simulink model "e4_tank_reactor_no_error_dyn"  (R2020a)
settings: Solver=FixedStepAuto  StartTime=0.0  StopTime=options.T_train  FixedStep=options.dt  RelTol=1e-3
PreLoadFcn:
  | load e4_PIDGainSchedExample.mat
model workspace (MAT data in the model file):
  op_snapshot1 : handle (value not decoded)
values from neighbouring files (symbols this model uses):
  C = [2 3 4 5 6 7 8 9]    [e4_PIDGainSchedExample.mat]
undefined symbols (not defined in the file or in its folder): Controllers, D, I, N, options, P, sigbuilder_block
libraries: neural x132, simulink x2, simulink_need_slupdate x1
(part 2 of 6)

== system e4_tank_reactor_no_error_dyn/NN/Layer 1/Delays 1 ==
  "p{1}" : Inport  PortDimensions=8
      mask Display: e = 0.06;c1 = [120 230 180]/255;c2 = ([120 230 180]+0)/(256+128);c3 = ([120 230 180]+128)/(256+128);patch([0 1 1 0],[0 0 1 1],c1);patch([0 1 1 1-e 1-e 0+e],[0 0 1 1-e 0+e 0+e],c2);patch([0 0 1 1-e 0+e 0+e],[0 1 1 1-e 1-e 0+e],c3);plot([0 1 1 0 0],[0 0 1 1 0]);
  mux : Mux  Inputs=1
      mask Display: e = 0.06;c1 = [120 150 230]/255;c2 = ([120 150 230]+0)/383;c3 = ([120 150 230]+128)/383;patch([0 1 1 0],[0 0 1 1],c1);patch([0 1 1 1-e 1-e 0+e],[0 0 1 1-e 0+e 0+e],c2);patch([0 0 1 1-e 0+e 0+e],[0 1 1 1-e 1-e 0+e],c3);plot([0 1 1 0 0],[0 0 1 1 0]);disp('Mux')
  "pd{1,1}" : Outport
      mask Display: e = 0.06;c1 = [120 230 180]/255;c2 = ([120 230 180]+0)/(256+128);c3 = ([120 230 180]+128)/(256+128);patch([0 1 1 0],[0 0 1 1],c1);patch([0 1 1 1-e 1-e 0+e],[0 0 1 1-e 0+e 0+e],c2);patch([0 0 1 1-e 0+e 0+e],[0 1 1 1-e 1-e 0+e],c3);plot([0 1 1 0 0],[0 0 1 1 0]);
  wires:
  "p{1}"/1 -> mux/1
  mux/1 -> "pd{1,1}"/1

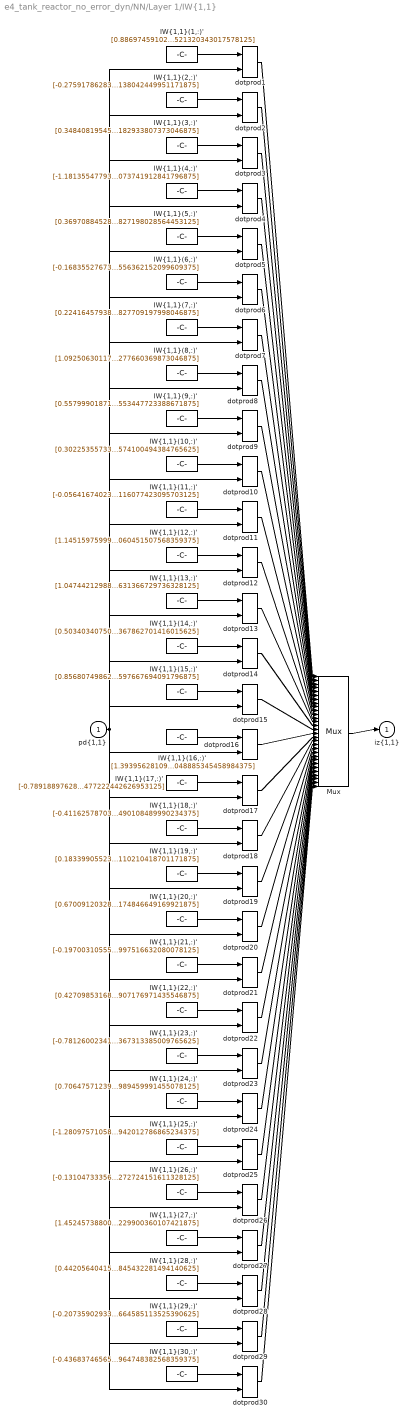
== system e4_tank_reactor_no_error_dyn/NN/Layer 1/IW{1,1} ==
  "pd{1,1}" : Inport  PortDimensions=8
      mask Display: e = 0.06;c1 = [120 230 180]/255;c2 = ([120 230 180]+0)/(256+128);c3 = ([120 230 180]+128)/(256+128);patch([0 1 1 0],[0 0 1 1],c1);patch([0 1 1 1-e 1-e 0+e],[0 0 1 1-e 0+e 0+e],c2);patch([0 0 1 1-e 0+e 0+e],[0 1 1 1-e 1-e 0+e],c3);plot([0 1 1 0 0],[0 0 1 1 0]);
  "IW{1,1}(1,:)'" : Constant  Value=[0.8869745910205413252924699918366968631744384765625;-0.003402523557962419502309625585212415899150073528289794921875;0.167531227865286069800276891328394412994384765625;0.10286305198869487298463099023138056509196758270263671875;-0.71703402880353894754961174839991144835948944091796875;-1.2912603656687069442199344848631881177425384521484375;0.9076414187719077375504639348946511745452880859375;0.424730339919138721871405550700728781521320343017578125]
      mask Display: e = 0.06;c1 = [120 150 230]/255;c2 = ([120 150 230]+0)/383;c3 = ([120 150 230]+128)/383;patch([0 1 1 0],[0 0 1 1],c1);patch([0 1 1 1-e 1-e 0+e],[0 0 1 1-e 0+e 0+e],c2);patch([0 0 1 1-e 0+e 0+e],[0 1 1 1-e 1-e 0+e],c3);plot([0 1 1 0 0],[0 0 1 1 0]);disp('Weights');
  "IW{1,1}(10,:)'" : Constant  Value=[0.302253557331712829903125339114922098815441131591796875;-1.9983086879888884990208453018567524850368499755859375;1.273941183184043257625717160408385097980499267578125;-1.018922795975827799708213206031359732151031494140625;2.4603325055853648706261083134450018405914306640625;-0.7659472736172781015540067528490908443927764892578125;-0.70371299108074636396992218578816391527652740478515625;0.12058703123603677076491891284604207612574100494384765625]
      mask Display: e = 0.06;c1 = [120 150 230]/255;c2 = ([120 150 230]+0)/383;c3 = ([120 150 230]+128)/383;patch([0 1 1 0],[0 0 1 1],c1);patch([0 1 1 1-e 1-e 0+e],[0 0 1 1-e 0+e 0+e],c2);patch([0 0 1 1-e 0+e 0+e],[0 1 1 1-e 1-e 0+e],c3);plot([0 1 1 0 0],[0 0 1 1 0]);disp('Weights');
  "IW{1,1}(11,:)'" : Constant  Value=[-0.056416740236481743853147463596542365849018096923828125;1.88817871488456301420910676824860274791717529296875;-0.2850288013275081855368853211984969675540924072265625;-0.60909058798571746873307120040408335626125335693359375;-1.1722779325389647286925765001797117292881011962890625;2.0040908100766454680297101731412112712860107421875;0.526873639458410369940111195319332182407379150390625;-0.92068711979477424467432911114883609116077423095703125]
      mask Display: e = 0.06;c1 = [120 150 230]/255;c2 = ([120 150 230]+0)/383;c3 = ([120 150 230]+128)/383;patch([0 1 1 0],[0 0 1 1],c1);patch([0 1 1 1-e 1-e 0+e],[0 0 1 1-e 0+e 0+e],c2);patch([0 0 1 1-e 0+e 0+e],[0 1 1 1-e 1-e 0+e],c3);plot([0 1 1 0 0],[0 0 1 1 0]);disp('Weights');
  "IW{1,1}(12,:)'" : Constant  Value=[1.14515975999364894022392036276869475841522216796875;-0.8542807808416206238888435109402053058147430419921875;1.066709048371362822393848546198569238185882568359375;0.377840995831276560412703702240833081305027008056640625;-1.020663060599571014819275660556741058826446533203125;-0.76558848030476622792406260487041436135768890380859375;0.7064741359778070606267874609329737722873687744140625;-0.6900660399931834998454860397032462060451507568359375]
      mask Display: e = 0.06;c1 = [120 150 230]/255;c2 = ([120 150 230]+0)/383;c3 = ([120 150 230]+128)/383;patch([0 1 1 0],[0 0 1 1],c1);patch([0 1 1 1-e 1-e 0+e],[0 0 1 1-e 0+e 0+e],c2);patch([0 0 1 1-e 0+e 0+e],[0 1 1 1-e 1-e 0+e],c3);plot([0 1 1 0 0],[0 0 1 1 0]);disp('Weights');
  "IW{1,1}(13,:)'" : Constant  Value=[1.04744212988422180643510728259570896625518798828125;-1.2053415482433142980056572923786006867885589599609375;-0.7225578173341260512785311220795847475528717041015625;-0.584831305619675223539388753124512732028961181640625;0.85698675098009668982257380775990895926952362060546875;-0.71145783550227281732958317661541514098644256591796875;-0.29166444409964886741448708562529645860195159912109375;-0.39113888775617511317506114210118539631366729736328125]
      mask Display: e = 0.06;c1 = [120 150 230]/255;c2 = ([120 150 230]+0)/383;c3 = ([120 150 230]+128)/383;patch([0 1 1 0],[0 0 1 1],c1);patch([0 1 1 1-e 1-e 0+e],[0 0 1 1-e 0+e 0+e],c2);patch([0 0 1 1-e 0+e 0+e],[0 1 1 1-e 1-e 0+e],c3);plot([0 1 1 0 0],[0 0 1 1 0]);disp('Weights');
  "IW{1,1}(14,:)'" : Constant  Value=[0.503403407506826994222137727774679660797119140625;-0.54357297238896240543226667796261608600616455078125;0.9874634317779336090126207636785693466663360595703125;0.033746523035958576886006454742528148926794528961181640625;-0.254811710231782118096788281036424450576305389404296875;0.86220415793024252071319324386422522366046905517578125;-0.83902536220982260051215462226537056267261505126953125;0.65023292766698459477225924274534918367862701416015625]
      mask Display: e = 0.06;c1 = [120 150 230]/255;c2 = ([120 150 230]+0)/383;c3 = ([120 150 230]+128)/383;patch([0 1 1 0],[0 0 1 1],c1);patch([0 1 1 1-e 1-e 0+e],[0 0 1 1-e 0+e 0+e],c2);patch([0 0 1 1-e 0+e 0+e],[0 1 1 1-e 1-e 0+e],c3);plot([0 1 1 0 0],[0 0 1 1 0]);disp('Weights');
  "IW{1,1}(15,:)'" : Constant  Value=[0.8568074986297740114338239436619915068149566650390625;-0.683506818415545058797988531296141445636749267578125;0.90244622966523613261102809701696969568729400634765625;-1.944132599731748012317211760091595351696014404296875;-0.58519215004215630049344554208801127970218658447265625;0.32903336516029302316610483103431761264801025390625;0.65754868586560533127993721791426651179790496826171875;-0.99959059893120627560136881584185175597667694091796875]
      mask Display: e = 0.06;c1 = [120 150 230]/255;c2 = ([120 150 230]+0)/383;c3 = ([120 150 230]+128)/383;patch([0 1 1 0],[0 0 1 1],c1);patch([0 1 1 1-e 1-e 0+e],[0 0 1 1-e 0+e 0+e],c2);patch([0 0 1 1-e 0+e 0+e],[0 1 1 1-e 1-e 0+e],c3);plot([0 1 1 0 0],[0 0 1 1 0]);disp('Weights');
  "IW{1,1}(16,:)'" : Constant  Value=[1.3939562810990129282373573005315847694873809814453125;1.0876382522002334685140567671624012291431427001953125;1.2710703159320801969300873679458163678646087646484375;-1.17347063100059489926252354052849113941192626953125;1.10341011023059021312064942321740090847015380859375;-0.316324187931432410092469353912747465074062347412109375;-0.7059769814258747278046257633832283318042755126953125;0.18481149462138490857654460342018865048885345458984375]
      mask Display: e = 0.06;c1 = [120 150 230]/255;c2 = ([120 150 230]+0)/383;c3 = ([120 150 230]+128)/383;patch([0 1 1 0],[0 0 1 1],c1);patch([0 1 1 1-e 1-e 0+e],[0 0 1 1-e 0+e 0+e],c2);patch([0 0 1 1-e 0+e 0+e],[0 1 1 1-e 1-e 0+e],c3);plot([0 1 1 0 0],[0 0 1 1 0]);disp('Weights');
  "IW{1,1}(17,:)'" : Constant  Value=[-0.78918897628251272191590715010534040629863739013671875;-0.69345544068538178539284899670747108757495880126953125;1.133331701461687490706253811367787420749664306640625;0.481227638616822994688249082173570059239864349365234375;1.394399245993624969486290865461342036724090576171875;0.7686987843847490342596984191914089024066925048828125;1.4818227960370886631125131316366605460643768310546875;-0.125485665132124613041497696031001396477222442626953125]
      mask Display: e = 0.06;c1 = [120 150 230]/255;c2 = ([120 150 230]+0)/383;c3 = ([120 150 230]+128)/383;patch([0 1 1 0],[0 0 1 1],c1);patch([0 1 1 1-e 1-e 0+e],[0 0 1 1-e 0+e 0+e],c2);patch([0 0 1 1-e 0+e 0+e],[0 1 1 1-e 1-e 0+e],c3);plot([0 1 1 0 0],[0 0 1 1 0]);disp('Weights');
  "IW{1,1}(18,:)'" : Constant  Value=[-0.4116257870393840168077304042526520788669586181640625;0.342402945255573187832709436406730674207210540771484375;0.6993052671719846014042332171811722218990325927734375;-0.04069640465013980856756603543544770218431949615478515625;0.060718970322058203603621251431832206435501575469970703125;-1.4315780103489730290533543666242621839046478271484375;0.746726210319609950971653233864344656467437744140625;-0.66922398088218082445877143982215784490108489990234375]
      mask Display: e = 0.06;c1 = [120 150 230]/255;c2 = ([120 150 230]+0)/383;c3 = ([120 150 230]+128)/383;patch([0 1 1 0],[0 0 1 1],c1);patch([0 1 1 1-e 1-e 0+e],[0 0 1 1-e 0+e 0+e],c2);patch([0 0 1 1-e 0+e 0+e],[0 1 1 1-e 1-e 0+e],c3);plot([0 1 1 0 0],[0 0 1 1 0]);disp('Weights');
  "IW{1,1}(19,:)'" : Constant  Value=[0.18339905523404398390852065858780406415462493896484375;1.5668662807207969223100008093751966953277587890625;-0.0268049996970174918275997555383582948707044124603271484375;0.07428825726819134056544413624578737653791904449462890625;-1.878491586774890809152793735847808420658111572265625;1.1916603403785341885878779066842980682849884033203125;1.672592346593904988338863404351286590099334716796875;-0.25617012853654486104204579532961361110210418701171875]
      mask Display: e = 0.06;c1 = [120 150 230]/255;c2 = ([120 150 230]+0)/383;c3 = ([120 150 230]+128)/383;patch([0 1 1 0],[0 0 1 1],c1);patch([0 1 1 1-e 1-e 0+e],[0 0 1 1-e 0+e 0+e],c2);patch([0 0 1 1-e 0+e 0+e],[0 1 1 1-e 1-e 0+e],c3);plot([0 1 1 0 0],[0 0 1 1 0]);disp('Weights');
  "IW{1,1}(2,:)'" : Constant  Value=[-0.27591786283207986318899429534212686121463775634765625;3.196411383092458091681464793509803712368011474609375;-1.0488445244355248942014213753282092511653900146484375;0.320146632870869807252489636084646917879581451416015625;-0.76571063454435772666073489745031110942363739013671875;-0.055011350027142767726839878150713047944009304046630859375;1.202802065550638843660635757260024547576904296875;-0.383647276981947171758946524278144352138042449951171875]
      mask Display: e = 0.06;c1 = [120 150 230]/255;c2 = ([120 150 230]+0)/383;c3 = ([120 150 230]+128)/383;patch([0 1 1 0],[0 0 1 1],c1);patch([0 1 1 1-e 1-e 0+e],[0 0 1 1-e 0+e 0+e],c2);patch([0 0 1 1-e 0+e 0+e],[0 1 1 1-e 1-e 0+e],c3);plot([0 1 1 0 0],[0 0 1 1 0]);disp('Weights');
  "IW{1,1}(20,:)'" : Constant  Value=[0.67009120328841598190905415322049520909786224365234375;-0.5515720185612804637997896861634217202663421630859375;-0.55267982206462662464474533408065326511859893798828125;-0.6448735709813189220795948131126351654529571533203125;0.06989978721913596426684733842193963937461376190185546875;-1.6288120176144247341909476745058782398700714111328125;0.779509281707432055696926909149624407291412353515625;1.310159712789221497786229519988410174846649169921875]
      mask Display: e = 0.06;c1 = [120 150 230]/255;c2 = ([120 150 230]+0)/383;c3 = ([120 150 230]+128)/383;patch([0 1 1 0],[0 0 1 1],c1);patch([0 1 1 1-e 1-e 0+e],[0 0 1 1-e 0+e 0+e],c2);patch([0 0 1 1-e 0+e 0+e],[0 1 1 1-e 1-e 0+e],c3);plot([0 1 1 0 0],[0 0 1 1 0]);disp('Weights');
  "IW{1,1}(21,:)'" : Constant  Value=[-0.1970031055596904445703643204979016445577144622802734375;-1.563987121958660964082810096442699432373046875;0.61059106825549569474986810746486298739910125732421875;1.031098034825259635027805416029877960681915283203125;0.56196026107034768859449513911386020481586456298828125;-1.9981853523962189722595894636469893157482147216796875;1.0888860789131200590418302454054355621337890625;-0.09361921948207392596419396113560651428997516632080078125]
      mask Display: e = 0.06;c1 = [120 150 230]/255;c2 = ([120 150 230]+0)/383;c3 = ([120 150 230]+128)/383;patch([0 1 1 0],[0 0 1 1],c1);patch([0 1 1 1-e 1-e 0+e],[0 0 1 1-e 0+e 0+e],c2);patch([0 0 1 1-e 0+e 0+e],[0 1 1 1-e 1-e 0+e],c3);plot([0 1 1 0 0],[0 0 1 1 0]);disp('Weights');
  "IW{1,1}(22,:)'" : Constant  Value=[0.427098531684761584248377630501636303961277008056640625;1.6076476568007012080130380127229727804660797119140625;-1.1014857891164815395512732720817439258098602294921875;0.36149790428804406960949791027815081179141998291015625;-0.248586804369456626506718066593748517334461212158203125;-0.69684275999031886072998531744815409183502197265625;-0.286841168321181394507135564708732999861240386962890625;0.422714361893740953046716413155081681907176971435546875]
      mask Display: e = 0.06;c1 = [120 150 230]/255;c2 = ([120 150 230]+0)/383;c3 = ([120 150 230]+128)/383;patch([0 1 1 0],[0 0 1 1],c1);patch([0 1 1 1-e 1-e 0+e],[0 0 1 1-e 0+e 0+e],c2);patch([0 0 1 1-e 0+e 0+e],[0 1 1 1-e 1-e 0+e],c3);plot([0 1 1 0 0],[0 0 1 1 0]);disp('Weights');
  "IW{1,1}(23,:)'" : Constant  Value=[-0.78126002341995481881298246662481687963008880615234375;-1.169284710329954624086212788824923336505889892578125;1.166017240859436920885627841926179826259613037109375;-0.8507388975249752238738665255368687212467193603515625;1.191358648701899891619859772617928683757781982421875;0.63702009366910161691777148007531650364398956298828125;0.74006431103171299579202013774192892014980316162109375;0.07772625224719166558973171277102665044367313385009765625]
      mask Display: e = 0.06;c1 = [120 150 230]/255;c2 = ([120 150 230]+0)/383;c3 = ([120 150 230]+128)/383;patch([0 1 1 0],[0 0 1 1],c1);patch([0 1 1 1-e 1-e 0+e],[0 0 1 1-e 0+e 0+e],c2);patch([0 0 1 1-e 0+e 0+e],[0 1 1 1-e 1-e 0+e],c3);plot([0 1 1 0 0],[0 0 1 1 0]);disp('Weights');
  "IW{1,1}(24,:)'" : Constant  Value=[0.7064757123964204854615900330827571451663970947265625;-1.18446852299836802302479554782621562480926513671875;0.8255008023140779638282538144267164170742034912109375;-1.131032706182091285285196136101149022579193115234375;-0.09862722601019034696090415081926039420068264007568359375;0.373718657230955653147930206614546477794647216796875;-0.238682435995127895100864634514437057077884674072265625;0.7577262920549394653590979942237026989459991455078125]
      mask Display: e = 0.06;c1 = [120 150 230]/255;c2 = ([120 150 230]+0)/383;c3 = ([120 150 230]+128)/383;patch([0 1 1 0],[0 0 1 1],c1);patch([0 1 1 1-e 1-e 0+e],[0 0 1 1-e 0+e 0+e],c2);patch([0 0 1 1-e 0+e 0+e],[0 1 1 1-e 1-e 0+e],c3);plot([0 1 1 0 0],[0 0 1 1 0]);disp('Weights');
  "IW{1,1}(25,:)'" : Constant  Value=[-1.2809757105870402948966102485428564250469207763671875;-0.82852550051283835319537729446892626583576202392578125;-0.32970505738248034877102554673911072313785552978515625;-0.279935523019308851733200071976170875132083892822265625;-1.055968298065763644189019032637588679790496826171875;0.704919073979582311295644103665836155414581298828125;-0.435018707569000684376447907197871245443820953369140625;0.7523081434708822623491641934379003942012786865234375]
      mask Display: e = 0.06;c1 = [120 150 230]/255;c2 = ([120 150 230]+0)/383;c3 = ([120 150 230]+128)/383;patch([0 1 1 0],[0 0 1 1],c1);patch([0 1 1 1-e 1-e 0+e],[0 0 1 1-e 0+e 0+e],c2);patch([0 0 1 1-e 0+e 0+e],[0 1 1 1-e 1-e 0+e],c3);plot([0 1 1 0 0],[0 0 1 1 0]);disp('Weights');
  "IW{1,1}(26,:)'" : Constant  Value=[-0.13104733356740727590050710205105133354663848876953125;2.32195529483453189101282987394370138645172119140625;-1.88567524333584923823536882991902530193328857421875;0.6858958644523547310001276855473406612873077392578125;-0.50214888361890064327752725148457102477550506591796875;-1.2241599972289074482745263594551943242549896240234375;0.34451596634661718621117643124307505786418914794921875;-0.1756704889982736716991240655261208303272724151611328125]
      mask Display: e = 0.06;c1 = [120 150 230]/255;c2 = ([120 150 230]+0)/383;c3 = ([120 150 230]+128)/383;patch([0 1 1 0],[0 0 1 1],c1);patch([0 1 1 1-e 1-e 0+e],[0 0 1 1-e 0+e 0+e],c2);patch([0 0 1 1-e 0+e 0+e],[0 1 1 1-e 1-e 0+e],c3);plot([0 1 1 0 0],[0 0 1 1 0]);disp('Weights');
  "IW{1,1}(27,:)'" : Constant  Value=[1.452457388008406180546217001392506062984466552734375;-1.172610436821962753839443394099362194538116455078125;-0.9004330461382306083351068082265555858612060546875;1.208817515055535363188710107351653277873992919921875;-1.5350383119922803576429259919677861034870147705078125;-1.2583216228706193273723101810901425778865814208984375;0.270644327489568625733085127649246715009212493896484375;-0.311405295052269159850055757488007657229900360107421875]
      mask Display: e = 0.06;c1 = [120 150 230]/255;c2 = ([120 150 230]+0)/383;c3 = ([120 150 230]+128)/383;patch([0 1 1 0],[0 0 1 1],c1);patch([0 1 1 1-e 1-e 0+e],[0 0 1 1-e 0+e 0+e],c2);patch([0 0 1 1-e 0+e 0+e],[0 1 1 1-e 1-e 0+e],c3);plot([0 1 1 0 0],[0 0 1 1 0]);disp('Weights');
  "IW{1,1}(28,:)'" : Constant  Value=[0.442056404152748660951743886471376754343509674072265625;0.2493526475618815518853210733141168020665645599365234375;0.1181239015107082568345475692694890312850475311279296875;-0.2496322625530794370174447749377577565610408782958984375;-1.4116755942211833829702527509653009474277496337890625;-0.244632780309239461491443989871186204254627227783203125;-0.92786848745628847101585279233404435217380523681640625;0.1302999051855696921453642289634444750845432281494140625]
      mask Display: e = 0.06;c1 = [120 150 230]/255;c2 = ([120 150 230]+0)/383;c3 = ([120 150 230]+128)/383;patch([0 1 1 0],[0 0 1 1],c1);patch([0 1 1 1-e 1-e 0+e],[0 0 1 1-e 0+e 0+e],c2);patch([0 0 1 1-e 0+e 0+e],[0 1 1 1-e 1-e 0+e],c3);plot([0 1 1 0 0],[0 0 1 1 0]);disp('Weights');
  "IW{1,1}(29,:)'" : Constant  Value=[-0.2073590293315980270794085527086281217634677886962890625;-1.261453485543998720430636240052990615367889404296875;0.417145317623059508349570023710839450359344482421875;0.4401304305971904806682459820876829326152801513671875;0.8012367360713794628424011534661985933780670166015625;0.93557485529794803813530279512633569538593292236328125;0.36557613193985805111196896177716553211212158203125;-1.159475113688609670958840069943107664585113525390625]
      mask Display: e = 0.06;c1 = [120 150 230]/255;c2 = ([120 150 230]+0)/383;c3 = ([120 150 230]+128)/383;patch([0 1 1 0],[0 0 1 1],c1);patch([0 1 1 1-e 1-e 0+e],[0 0 1 1-e 0+e 0+e],c2);patch([0 0 1 1-e 0+e 0+e],[0 1 1 1-e 1-e 0+e],c3);plot([0 1 1 0 0],[0 0 1 1 0]);disp('Weights');
  "IW{1,1}(3,:)'" : Constant  Value=[0.348408195456650859878067194586037658154964447021484375;0.13128979584945010827823352883569896221160888671875;-1.2462763128456197936344551635556854307651519775390625;0.8373497908577769432980630881502293050289154052734375;0.680450778974826864242686497163958847522735595703125;-0.7039887459854632378863925623591057956218719482421875;-1.1005637181368499444289454913814552128314971923828125;-0.666422487535424323823463055305182933807373046875]
      mask Display: e = 0.06;c1 = [120 150 230]/255;c2 = ([120 150 230]+0)/383;c3 = ([120 150 230]+128)/383;patch([0 1 1 0],[0 0 1 1],c1);patch([0 1 1 1-e 1-e 0+e],[0 0 1 1-e 0+e 0+e],c2);patch([0 0 1 1-e 0+e 0+e],[0 1 1 1-e 1-e 0+e],c3);plot([0 1 1 0 0],[0 0 1 1 0]);disp('Weights');
  "IW{1,1}(30,:)'" : Constant  Value=[-0.43683746565477676870870027414639480412006378173828125;0.414885905669120591543475029538967646658420562744140625;0.71161051729680802058197741644107736647129058837890625;-0.0266920397314014158640649299059077748097479343414306640625;-1.3723826044633893328494878005585633218288421630859375;-0.4296181668357093030863325111567974090576171875;-1.212987357728822157554304794757626950740814208984375;-0.67853804582980214998855217345408163964748382568359375]
      mask Display: e = 0.06;c1 = [120 150 230]/255;c2 = ([120 150 230]+0)/383;c3 = ([120 150 230]+128)/383;patch([0 1 1 0],[0 0 1 1],c1);patch([0 1 1 1-e 1-e 0+e],[0 0 1 1-e 0+e 0+e],c2);patch([0 0 1 1-e 0+e 0+e],[0 1 1 1-e 1-e 0+e],c3);plot([0 1 1 0 0],[0 0 1 1 0]);disp('Weights');
  "IW{1,1}(4,:)'" : Constant  Value=[-1.1813554779349157985990359520656056702136993408203125;1.3081343050477116651819642356713302433490753173828125;0.1111861520282881043986122904243529774248600006103515625;0.302078564819876493885431045782752335071563720703125;-1.215049696649854293895032242289744317531585693359375;-0.339238609197104412640300097336876206099987030029296875;-0.146943201435645598440515868787770159542560577392578125;0.19192274869351688693086543935351073741912841796875]
      mask Display: e = 0.06;c1 = [120 150 230]/255;c2 = ([120 150 230]+0)/383;c3 = ([120 150 230]+128)/383;patch([0 1 1 0],[0 0 1 1],c1);patch([0 1 1 1-e 1-e 0+e],[0 0 1 1-e 0+e 0+e],c2);patch([0 0 1 1-e 0+e 0+e],[0 1 1 1-e 1-e 0+e],c3);plot([0 1 1 0 0],[0 0 1 1 0]);disp('Weights');
  "IW{1,1}(5,:)'" : Constant  Value=[0.369708845289564658198600000105216167867183685302734375;-1.1370366447060458181539388533565215766429901123046875;1.3116044914015230204995532403700053691864013671875;-0.1427314167325453853063521592048346064984798431396484375;0.88665021491913320605959825115860439836978912353515625;0.87832821946413108804563307785429060459136962890625;-0.304666739704737621341479325565160252153873443603515625;-0.33909715679392082865462043628212995827198028564453125]
      mask Display: e = 0.06;c1 = [120 150 230]/255;c2 = ([120 150 230]+0)/383;c3 = ([120 150 230]+128)/383;patch([0 1 1 0],[0 0 1 1],c1);patch([0 1 1 1-e 1-e 0+e],[0 0 1 1-e 0+e 0+e],c2);patch([0 0 1 1-e 0+e 0+e],[0 1 1 1-e 1-e 0+e],c3);plot([0 1 1 0 0],[0 0 1 1 0]);disp('Weights');
  "IW{1,1}(6,:)'" : Constant  Value=[-0.1683552767320385668003979162676841951906681060791015625;1.4155439500628876903220998428878374397754669189453125;-0.3049936648618356560547226763446815311908721923828125;-0.1808735587972198910478027755743823945522308349609375;-0.93949487207675286271069126087240874767303466796875;-0.98517475915990926349508072235039435327053070068359375;0.52147568646198638742106368226814083755016326904296875;-0.4491059618427362121195756117231212556362152099609375]
      mask Display: e = 0.06;c1 = [120 150 230]/255;c2 = ([120 150 230]+0)/383;c3 = ([120 150 230]+128)/383;patch([0 1 1 0],[0 0 1 1],c1);patch([0 1 1 1-e 1-e 0+e],[0 0 1 1-e 0+e 0+e],c2);patch([0 0 1 1-e 0+e 0+e],[0 1 1 1-e 1-e 0+e],c3);plot([0 1 1 0 0],[0 0 1 1 0]);disp('Weights');
  "IW{1,1}(7,:)'" : Constant  Value=[0.2241645793824775523273018507097731344401836395263671875;1.342167864111561303985808990546502172946929931640625;-0.0032931951292033919721780055311910473392345011234283447265625;-0.52511153598029525202406375683494843542575836181640625;-1.6807771985161521488549851710558868944644927978515625;0.5566622950019202153981723313336260616779327392578125;0.719828629925344021245336989522911608219146728515625;0.10582018054103141391220077593970927409827709197998046875]
      mask Display: e = 0.06;c1 = [120 150 230]/255;c2 = ([120 150 230]+0)/383;c3 = ([120 150 230]+128)/383;patch([0 1 1 0],[0 0 1 1],c1);patch([0 1 1 1-e 1-e 0+e],[0 0 1 1-e 0+e 0+e],c2);patch([0 0 1 1-e 0+e 0+e],[0 1 1 1-e 1-e 0+e],c3);plot([0 1 1 0 0],[0 0 1 1 0]);disp('Weights');
  "IW{1,1}(8,:)'" : Constant  Value=[1.0925063011756928066375849084579385817050933837890625;-0.57675375136482198712428726139478385448455810546875;-0.4110002600985167564573430354357697069644927978515625;0.459619928994233040153716274289763532578945159912109375;-0.97175270511539835194270153806428425014019012451171875;0.48179036288909216079190400705556385219097137451171875;0.62766837769450789519254385595559142529964447021484375;-1.264282084455540466905176799627952277660369873046875]
      mask Display: e = 0.06;c1 = [120 150 230]/255;c2 = ([120 150 230]+0)/383;c3 = ([120 150 230]+128)/383;patch([0 1 1 0],[0 0 1 1],c1);patch([0 1 1 1-e 1-e 0+e],[0 0 1 1-e 0+e 0+e],c2);patch([0 0 1 1-e 0+e 0+e],[0 1 1 1-e 1-e 0+e],c3);plot([0 1 1 0 0],[0 0 1 1 0]);disp('Weights');
  "IW{1,1}(9,:)'" : Constant  Value=[0.55799901871459145485943054154631681740283966064453125;-0.2030729847481355931915203427706728689372539520263671875;1.198759729689530484364468065905384719371795654296875;-0.77633171495453290322785733224009163677692413330078125;0.1732250078450238983673870052371057681739330291748046875;-0.41468434699252465502894438031944446265697479248046875;-0.6686192894460825097979750353260897099971771240234375;0.039408810987360758104625091391426394693553447723388671875]
      mask Display: e = 0.06;c1 = [120 150 230]/255;c2 = ([120 150 230]+0)/383;c3 = ([120 150 230]+128)/383;patch([0 1 1 0],[0 0 1 1],c1);patch([0 1 1 1-e 1-e 0+e],[0 0 1 1-e 0+e 0+e],c2);patch([0 0 1 1-e 0+e 0+e],[0 1 1 1-e 1-e 0+e],c3);plot([0 1 1 0 0],[0 0 1 1 0]);disp('Weights');
  Mux : Mux  Inputs=30
      mask Display: e = 0.06;c1 = [120 150 230]/255;c2 = ([120 150 230]+0)/383;c3 = ([120 150 230]+128)/383;patch([0 1 1 0],[0 0 1 1],c1);patch([0 1 1 1-e 1-e 0+e],[0 0 1 1-e 0+e 0+e],c2);patch([0 0 1 1-e 0+e 0+e],[0 1 1 1-e 1-e 0+e],c3);plot([0 1 1 0 0],[0 0 1 1 0]);disp('Mux');
  dotprod{1..30} (30 alike) : neural/Weight Functions/dotprod
  "iz{1,1}" : Outport
      mask Display: e = 0.06;c1 = [120 230 180]/255;c2 = ([120 230 180]+0)/(256+128);c3 = ([120 230 180]+128)/(256+128);patch([0 1 1 0],[0 0 1 1],c1);patch([0 1 1 1-e 1-e 0+e],[0 0 1 1-e 0+e 0+e],c2);patch([0 0 1 1-e 0+e 0+e],[0 1 1 1-e 1-e 0+e],c3);plot([0 1 1 0 0],[0 0 1 1 0]);
  wires:
  "IW{1,1}(1,:)'"/1 -> dotprod1/1
  "pd{1,1}"/1 -> dotprod1/2, dotprod2/2, dotprod3/2, dotprod4/2, dotprod5/2, dotprod6/2, dotprod7/2, dotprod8/2, dotprod9/2, dotprod10/2, dotprod11/2, dotprod12/2, dotprod13/2, dotprod14/2, dotprod15/2, dotprod16/2, dotprod17/2, dotprod18/2, dotprod19/2, dotprod20/2, dotprod21/2, dotprod22/2, dotprod23/2, dotprod24/2, dotprod25/2, dotprod26/2, dotprod27/2, dotprod28/2, dotprod29/2, dotprod30/2
  dotprod1/1 -> Mux/1
  "IW{1,1}(2,:)'"/1 -> dotprod2/1
  dotprod2/1 -> Mux/2
  "IW{1,1}(3,:)'"/1 -> dotprod3/1
  dotprod3/1 -> Mux/3
  "IW{1,1}(4,:)'"/1 -> dotprod4/1
  dotprod4/1 -> Mux/4
  "IW{1,1}(5,:)'"/1 -> dotprod5/1
  dotprod5/1 -> Mux/5
  "IW{1,1}(6,:)'"/1 -> dotprod6/1
  dotprod6/1 -> Mux/6
  "IW{1,1}(7,:)'"/1 -> dotprod7/1
  dotprod7/1 -> Mux/7
  "IW{1,1}(8,:)'"/1 -> dotprod8/1
  dotprod8/1 -> Mux/8
  "IW{1,1}(9,:)'"/1 -> dotprod9/1
  dotprod9/1 -> Mux/9
  "IW{1,1}(10,:)'"/1 -> dotprod10/1
  dotprod10/1 -> Mux/10
  "IW{1,1}(11,:)'"/1 -> dotprod11/1
  dotprod11/1 -> Mux/11
  "IW{1,1}(12,:)'"/1 -> dotprod12/1
  dotprod12/1 -> Mux/12
  "IW{1,1}(13,:)'"/1 -> dotprod13/1
  dotprod13/1 -> Mux/13
  "IW{1,1}(14,:)'"/1 -> dotprod14/1
  dotprod14/1 -> Mux/14
  "IW{1,1}(15,:)'"/1 -> dotprod15/1
  dotprod15/1 -> Mux/15
  "IW{1,1}(16,:)'"/1 -> dotprod16/1
  dotprod16/1 -> Mux/16
  "IW{1,1}(17,:)'"/1 -> dotprod17/1
  dotprod17/1 -> Mux/17
  "IW{1,1}(18,:)'"/1 -> dotprod18/1
  dotprod18/1 -> Mux/18
  "IW{1,1}(19,:)'"/1 -> dotprod19/1
  dotprod19/1 -> Mux/19
  "IW{1,1}(20,:)'"/1 -> dotprod20/1
  dotprod20/1 -> Mux/20
  "IW{1,1}(21,:)'"/1 -> dotprod21/1
  dotprod21/1 -> Mux/21
  "IW{1,1}(22,:)'"/1 -> dotprod22/1
  dotprod22/1 -> Mux/22
  "IW{1,1}(23,:)'"/1 -> dotprod23/1
  dotprod23/1 -> Mux/23
  "IW{1,1}(24,:)'"/1 -> dotprod24/1
  dotprod24/1 -> Mux/24
  "IW{1,1}(25,:)'"/1 -> dotprod25/1
  dotprod25/1 -> Mux/25
  "IW{1,1}(26,:)'"/1 -> dotprod26/1
  dotprod26/1 -> Mux/26
  "IW{1,1}(27,:)'"/1 -> dotprod27/1
  dotprod27/1 -> Mux/27
  "IW{1,1}(28,:)'"/1 -> dotprod28/1
  dotprod28/1 -> Mux/28
  "IW{1,1}(29,:)'"/1 -> dotprod29/1
  dotprod29/1 -> Mux/29
  "IW{1,1}(30,:)'"/1 -> dotprod30/1
  dotprod30/1 -> Mux/30
  Mux/1 -> "iz{1,1}"/1

== system e4_tank_reactor_no_error_dyn/NN/Layer 2/Delays 1 ==
  "p{2}" : Inport  PortDimensions=30
      mask Display: e = 0.06;c1 = [120 230 180]/255;c2 = ([120 230 180]+0)/(256+128);c3 = ([120 230 180]+128)/(256+128);patch([0 1 1 0],[0 0 1 1],c1);patch([0 1 1 1-e 1-e 0+e],[0 0 1 1-e 0+e 0+e],c2);patch([0 0 1 1-e 0+e 0+e],[0 1 1 1-e 1-e 0+e],c3);plot([0 1 1 0 0],[0 0 1 1 0]);
  mux : Mux  Inputs=1
      mask Display: e = 0.06;c1 = [120 150 230]/255;c2 = ([120 150 230]+0)/383;c3 = ([120 150 230]+128)/383;patch([0 1 1 0],[0 0 1 1],c1);patch([0 1 1 1-e 1-e 0+e],[0 0 1 1-e 0+e 0+e],c2);patch([0 0 1 1-e 0+e 0+e],[0 1 1 1-e 1-e 0+e],c3);plot([0 1 1 0 0],[0 0 1 1 0]);disp('Mux')
  "pd{2,1}" : Outport
      mask Display: e = 0.06;c1 = [120 230 180]/255;c2 = ([120 230 180]+0)/(256+128);c3 = ([120 230 180]+128)/(256+128);patch([0 1 1 0],[0 0 1 1],c1);patch([0 1 1 1-e 1-e 0+e],[0 0 1 1-e 0+e 0+e],c2);patch([0 0 1 1-e 0+e 0+e],[0 1 1 1-e 1-e 0+e],c3);plot([0 1 1 0 0],[0 0 1 1 0]);
  wires:
  "p{2}"/1 -> mux/1
  mux/1 -> "pd{2,1}"/1
